simulink model "Pitch_Ap_testHarness"  (R2012b)
settings: Solver=FixedStepDiscrete  SolverMode=SingleTasking  StartTime=0  StopTime=0.25  FixedStep=0.025  RelTol=1e-3
model workspace (MAT data in the model file):
  dispGain = [3707764736; 2; 1; 1; 1; 1]
  intGain = [3707764736; 2; 1; 1; 2; 1]
  rateGain = [3707764736; 2; 1; 1; 3; 1]
undefined symbols (not defined in the file): sigbuilder_block
libraries: simulink x1
settings Model: SldvGeneratedHarnessModel=TestUnitModel=Pitch_Ap|  RecordCoverage=on  CovSaveName=covdata_pitchAP  CovMetricSettings=dcmoe  CovHTMLOptions=-aTS=1 -bRG=1 -bTC=0 -hTR=0 -nFC=0 -scm=1 -bcm=1  CovCumulativeVarName=covCumulativeData_pitchAP  CovCumulativeReport=on  CovReportOnPause=off  CovModelRefEnable=on  CovExternalEMLEnable=on  Creator=bpotter  LastModifiedBy=klindqvi
settings DataIOCC: LimitDataPoints=off  SaveFormat=StructureWithTime  SignalLoggingSaveFormat=ModelDataLogs  SaveOutput=off  DSMLogging=off  SaveTime=off  SignalLoggingName=logsOut
settings OptimizationCC: BlockReduction=off  InlineParams=on  UseIntDivNetSlope=on  InlineInvariantSignals=on  EnhancedBackFolding=on  ExpressionFolding=off  EnableMemcpy=off  PassReuseOutputArgsAs=Individual arguments  StateBitsets=on  DataBitsets=on  ZeroExternalMemoryAtStartup=off  ZeroInternalMemoryAtStartup=off  InitFltsAndDblsToZero=on  EfficientFloat2IntCast=on  EfficientMapNaN2IntZero=off  OptimizeModelRefInitCode=on  MaxStackSize=inf
settings DebuggingCC: SignalInfNanChecking=error  ReadBeforeWriteMsg=EnableAllAsError  WriteAfterWriteMsg=EnableAllAsError  WriteAfterReadMsg=EnableAllAsError  AlgebraicLoopMsg=error  ArtificialAlgebraicLoopMsg=error  SaveWithDisabledLinksMsg=error  SaveWithParameterizedLinksMsg=error  UnderspecifiedInitializationDetection=Simplified  BlockPriorityViolationMsg=error  MaxConsecutiveZCsMsg=warning  SolverPrmCheckMsg=error  InheritedTsInSrcMsg=none  DiscreteInheritContinuousMsg=error  SingleTaskRateTransMsg=error  TasksWithSamePriorityMsg=error  SigSpecEnsureSampleTimeMsg=error  CheckMatrixSingularityMsg=error  IntegerOverflowMsg=none  ParameterUnderflowMsg=error  ParameterPrecisionLossMsg=error  ParameterTunabilityLossMsg=error  UnderSpecifiedDataTypeMsg=error  UnnecessaryDatatypeConvMsg=warning  VectorMatrixConversionMsg=error  SignalLabelMismatchMsg=error  UnconnectedInputMsg=error  UnconnectedOutputMsg=error  UnconnectedLineMsg=error  SFcnCompatibilityMsg=error  UniqueDataStoreMsg=error  BusObjectLabelMismatch=error  RootOutportRequireBusObject=error  AssertControl=DisableAll  ModelReferenceIOMsg=error  ModelReferenceVersionMismatchMessage=warning  ModelReferenceIOMismatchMessage=error  UnknownTsInhSupMsg=error  ModelReferenceDataLoggingMessage=error  ModelReferenceExtraNoncontSigs=none  StrictBusMsg=ErrorOnBusTreatedAsVector  BusNameAdapt=ErrorWithoutRepair  NonBusSignalsTreatedAsBus=error
settings HardwareCC: ProdIntDivRoundTo=Zero  ProdEndianess=LittleEndian  ProdHWDeviceType=Specified
settings ModelReferenceCC: UpdateModelReferenceTargets=AssumeUpToDate  CheckModelReferenceTargetMessage=none
settings RTWCC: SystemTargetFile=ert.tlc  TemplateMakefile=ert_default_tmf  Description=Embedded Coder  GenerateReport=on  RTWVerbose=off  ProcessScript=ert_make_rtw_hook  IncludeHyperlinkInReport=on  GenerateTraceInfo=on  GenerateTraceReport=on  GenerateTraceReportSl=on  GenerateTraceReportSf=on  GenerateTraceReportEml=on  GenerateCodeMetricsReport=on
settings CodeAppCC: ForceParamTrailComments=on  IgnoreCustomStorageClasses=off  IgnoreTestpoints=on  SimulinkDataObjDesc=on  MangleLength=4  CustomSymbolStrGlobalVar=$N$M  CustomSymbolStrType=$N$M  CustomSymbolStrFcn=$N$M$F  CustomSymbolStrMacro=$N$M  InsertBlockDesc=on  ReqsInCode=on
settings ERTTargetCC: CodeReplacementLibrary=ANSI_C  UtilityFuncGeneration=Shared location  MultiwordLength=2048  GenerateSampleERTMain=on  IncludeMdlTerminateFcn=off  GeneratePreprocessorConditionals=Disable all  SuppressErrorStatus=on  SupportAbsoluteTime=off  MultiInstanceERTCode=on  SupportNonFinite=off  SupportComplex=off  ParenthesesLevel=Maximum  InlinedParameterPlacement=NonHierarchical  ERTCustomFileTemplate=example_file_process.tlc  ERTFilePackagingFormat=CompactWithDataFile  PreserveExpressionOrder=on  PreserveIfCondition=on  ConvertIfToSwitch=off  SuppressUnreachableDefaultCases=off

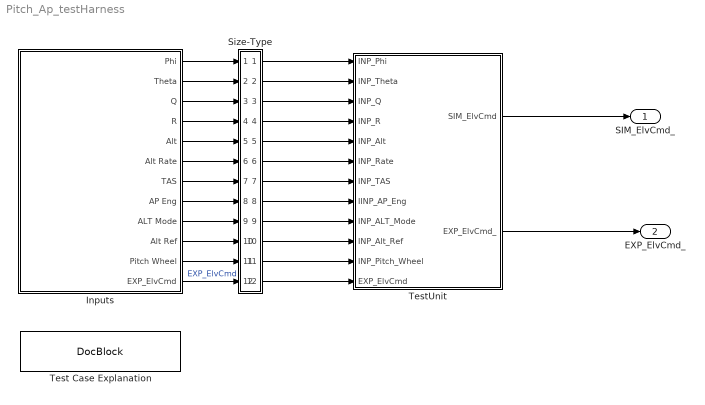
== system Pitch_Ap_testHarness ==
  Inputs : Subsystem  Tag=STV Subsys  LoadFcn=sigbuilder_block('load');  StartFcn=sigbuilder_block('start');  StopFcn=sigbuilder_block('stop');  ClipboardFcn=sigbuilder_block('clipboard');  mask(Sigbuilder block){}
      mask init:
      | if ~strcmp(get_param(bdroot(gcb),'SimulationStatus'),'stopped'),tuvar = sigbuilder_block('maskInit'); end
      settings: CopyFcn=sigbuilder_block('copy');  DeleteFcn=sigbuilder_block('delete');  ModelCloseFcn=sigbuilder_block('modelClose');  PreSaveFcn=sigbuilder_block('preSave');  PauseFcn=sigbuilder_block('pause');  ContinueFcn=sigbuilder_block('continue');  NameChangeFcn=sigbuilder_block('namechange');  OpenFcn=sigbuilder_block('open',[18 174 755.25 438 ]);  CloseFcn=sigbuilder_block('close');
      mask Display: plot(0, 0, 100, 100,[2, 2, 32, 32, 2], [68, 8, 8, 68, 68],[32, 2], [38, 38], [32, 19, 2],[53, 60, 44], [32, 17, 17, 2],[16, 16, 31, 31]);txt = getActiveGroup(gcbh);text(2, 100, txt,'verticalAlignment', 'top');
  Size-Type : Subsystem
  Test Case Explanation : simulink/Model-Wide Utilities/DocBlock  DocumentType=Text
      content=|
      | Test Case 1 (38 Objectives)
      | 	Parameter values:
      |
      | 	1. Altitude Mode/Rate Limiter/Saturation Dynamic/Switch - logical trigger input false (output is from 3rd input port) @ T=0.08
      | 	2. Altitude Mode/Rate Limiter/Saturation Dynamic/Switch - logical trigger input true (output is from 1st input port) @ T=0.15
      | 	3. Attitude_Controller/Cmd Limit - input > lower limit T @ T=0.05
      | 	4. Attitude_Controller/Cmd Limit - input >= upper limit F @ T=0.05
      | 	5. Attitude_Controller/LevelResetIntegrator/Saturation - input > lower limit T @ T=0.05
      | 	6. Attitude_Controller/LevelResetIntegrator/Saturation - input >= upper limit F @ T=0.05
      | 	7. Pitch Reference/Latch Theta/Enable - logical trigger input false (output is from 3rd input port) @ T=0.05
      | 	8. Pitch Reference/Latch Theta/Enable - logical trigger input true (output is from 1st input port) @ T=0.00
      | 	9. Altitude Mode/Rate Limiter/Saturation Dynamic/Switch2 - logical trigger input false (output is from 3rd input port) @ T=0.08
      | 	10. Altitude Mode/Rate Limiter/Saturation Dynamic/Switch2 - logical trigger input true (output is from 1st input port) @ T=0.00
      | 	11. Altitude Mode/Switch - logical trigger input false (output is from 3rd input port) @ T=0.10
      | 	12. Altitude Mode/Switch - logical trigger input true (output is from 1st input port) @ T=0.00
      | 	13. Attitude_Controller/LevelResetIntegrator/Switch1 - logical trigger input false (output is from 3rd input port) @ T=0.05
      | 	14. Attitude_Controller/LevelResetIntegrator/Switch1 - logical trigger input true (output is from 1st input port) @ T=0.00
      | 	15. Eng switch - logical trigger input false (output is from 3rd input port) @ T=0.00
      | 	16. Eng switch - logical trigger input true (output is from 1st input port) @ T=0.05
      | 	17. Mode switch - logical trigger input false (output is from 3rd input port) @ T=0.00
      | 	18. Mode switch - logical trigger input true (output is from 1st input port) @ T=0.10
      | 	19. Pitch Reference/Not engaged - Logic: input port 1 T @ T=0.05
      | 	20. Pitch Reference/Not engaged - Logic: input port 1 F @ T=0.00
      | 	21. Altitude Mode/Integrator - Reset F @ T=0.13
      | 	22. Altitude Mode/Integrator - Reset T @ T=0.03
      | 	23. Altitude Mode/Integrator - integration result <= lower limit F @ T=0.05
      | 	24. Altitude Mode/Integrator - integration result <= lower limit T @ T=0.00
      | 	25. Altitude Mode/Integrator - integration result >= upper limit F @ T=0.00
      | 	26. Altitude Mode/Integrator - integration result >= upper limit T @ T=0.18
      | 	27. Altitude Mode/Not ALT - Logic: input port 1 T @ T=0.10
      | 	28. Altitude Mode/Not ALT - Logic: input port 1 F @ T=0.00
      | 	29. Attitude_Controller/LevelResetIntegrator/Switch - logical trigger input false (output is from 3rd input port) @ T=0.05
      | 	30. Attitude_Controller/LevelResetIntegrator/Switch - logical trigger input true (output is from 1st input port) @ T=0.00
      | 	31. Attitude_Controller/Rate Limit - input > lower limit T @ T=0.00
      | 	32. Attitude_Controller/Rate Limit - input >= upper limit F @ T=0.00
      | 	33. Attitude_Controller/Rate Limit - input >= upper limit T @ T=0.18
      | 	34. Attitude_Controller/Disp Limit - input > lower limit T @ T=0.00
      | 	35. Attitude_Controller/Disp Limit - input >= upper limit F @ T=0.00
      | 	36. Attitude_Controller/Disp Limit - input >= upper limit T @ T=0.20
      | 	37. Attitude_Controller/Not engaged - Logic: input port 1 T @ T=0.05
      | 	38. Attitude_Controller/Not engaged - Logic: input port 1 F @ T=0.00
      |
      | Test Case 2 (3 Objectives)
      | 	Parameter values:
      |
      | 	1. Attitude_Controller/Cmd Limit - input > lower limit F @ T=0.00
      | 	2. Attitude_Controller/Rate Limit - input > lower limit F @ T=0.00
      | 	3. Attitude_Controller/Disp Limit - input > lower limit F @ T=0.03
      |
      | Test Case 3 (1 Objectives)
      | 	Parameter values:
      |
      | 	1. Attitude_Controller/Cmd Limit - input >= upper limit T @ T=0.00
  TestUnit : Subsystem
  SIM_ElvCmd_ : Outport  OutDataTypeStr=double  PortDimensions=1  SampleTime=1/40
  EXP_ElvCmd_ : Outport  Port=2  OutDataTypeStr=double  PortDimensions=1  SampleTime=1/40
  wires:
  Inputs/1(Phi) -> Size-Type/1(In1)
  Inputs/2(Theta) -> Size-Type/2(In2)
  Inputs/3(Q) -> Size-Type/3(In3)
  Inputs/4(R) -> Size-Type/4(In4)
  Inputs/5(Alt) -> Size-Type/5(In5)
  Inputs/6(Alt Rate) -> Size-Type/6(In6)
  Inputs/7(TAS) -> Size-Type/7(In7)
  Inputs/8(AP Eng) -> Size-Type/8(In8)
  Inputs/9(ALT Mode) -> Size-Type/9(In9)
  Inputs/10(Alt Ref) -> Size-Type/10(In10)
  Inputs/11("Pitch Wheel ") -> Size-Type/11(In11)
  Size-Type/1(Out1) -> TestUnit/1(INP_Phi)
  Size-Type/2(Out2) -> TestUnit/2(INP_Theta)
  Size-Type/3(Out3) -> TestUnit/3(INP_Q)
  Size-Type/4(Out4) -> TestUnit/4(INP_R)
  Size-Type/5(Out5) -> TestUnit/5(INP_Alt)
  Size-Type/6(Out6) -> TestUnit/6(INP_Rate)
  Size-Type/7(Out7) -> TestUnit/7(INP_TAS)
  Size-Type/8(Out8) -> TestUnit/8(IINP_AP_Eng)
  Size-Type/9(Out9) -> TestUnit/9(INP_ALT_Mode)
  Size-Type/10(Out10) -> TestUnit/10(INP_Alt_Ref)
  Size-Type/11(Out11) -> TestUnit/11(INP_Pitch_Wheel)
  TestUnit/1(SIM_ElvCmd) -> SIM_ElvCmd_/1
  TestUnit/2(EXP_ElvCmd_) -> EXP_ElvCmd_/1
  Inputs/12(EXP_ElvCmd) -> Size-Type/12(In12)  "EXP_ElvCmd"
  Size-Type/12(Out12) -> TestUnit/12(EXP_ElvCmd)

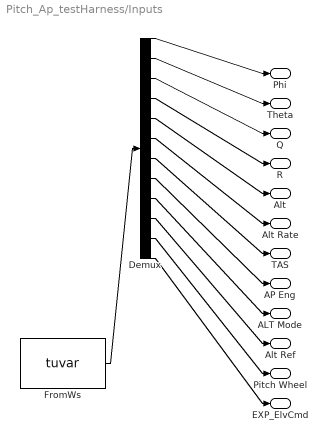
== system Pitch_Ap_testHarness/Inputs ==
  Demux : Demux  Tag=STV Demux  Outputs=12
  FromWs : FromWorkspace  Tag=STV FromWs  VariableName=tuvar  SampleTime=0
      SigBuilderData=|
      | dataSet(1).timeRange = [0 0.25]
      | dataSet(1).name = 'Test Case 1'
      | dataSet(2).timeRange = [0 0.075]
      | dataSet(2).name = 'Test Case 2'
      | dataSet(3).timeRange = [0 0.05]
      | dataSet(3).name = 'Test Case 3'
      | sbobj.Name = 'Signal Builder'
      | sbobj.Groups(1).Name = 'Test Case 1'
      | sbobj.Groups(1).Signals(1).Name = 'Phi'
      | sbobj.Groups(1).Signals(1).XData = [0 0.05 0.05 0.1 0.15 0.15 0.175 0.175 0.2 0.2 0.225 0.25]
      | sbobj.Groups(1).Signals(1).YData = [-8.54927 -8.54927 0 0 0 -6.7752 -6.7752 -1.37522 -1.37522 0 0 0]
      | sbobj.Groups(1).Signals(2).Name = 'Theta'
      | sbobj.Groups(1).Signals(2).XData = [0 0.05 0.05 0.1 0.1 0.15 0.15 0.175 0.175 0.2 0.2 0.225 0.225 0.25]
      | sbobj.Groups(1).Signals(2).YData = [0.8763 0.8763 0 0 0 0 1.88631 1.88631 -7.95353 -7.95353 0 0 0 0]
      | sbobj.Groups(1).Signals(3).Name = 'Q'
      | sbobj.Groups(1).Signals(3).XData = [0 0.05 0.05 0.1 0.1 0.15 0.15 0.175 0.175 0.2 0.2 0.225 0.225 0.25]
      | sbobj.Groups(1).Signals(3).YData = [9.81417 9.81417 0 0 0 0 4.66234 4.66234 3.21637 3.21637 0 0 0 0]
      | sbobj.Groups(1).Signals(4).Name = 'R'
      | sbobj.Groups(1).Signals(4).XData = [0 0.05 0.05 0.1 0.1 0.15 0.15 0.175 0.175 0.2 0.2 0.225 0.225 0.25]
      | sbobj.Groups(1).Signals(4).YData = [-5.97411 -5.97411 0 0 0 0 -2.73996 -2.73996 2.52191 2.52191 0 0 0 0]
      | sbobj.Groups(1).Signals(5).Name = 'Alt'
      | sbobj.Groups(1).Signals(5).XData = [0 0.05 0.05 0.1 0.1 0.15 0.15 0.175 0.175 0.2 0.2 0.225 0.225 0.25]
      | sbobj.Groups(1).Signals(5).YData = [3.08094 3.08094 0 0 0 0 -9.43223 -9.43223 -6.0138 -6.0138 0 0 0 0]
      | sbobj.Groups(1).Signals(6).Name = 'Alt Rate'
      | sbobj.Groups(1).Signals(6).XData = [0 0.05 0.05 0.1 0.1 0.15 0.15 0.175 0.175 0.2 0.2 0.225 0.225 0.25]
      | sbobj.Groups(1).Signals(6).YData = [2.41404 2.41404 0 0 0 0 -3.30183 -3.30183 5.00647 5.00647 0 0 0 0]
      | sbobj.Groups(1).Signals(7).Name = 'TAS'
      | sbobj.Groups(1).Signals(7).XData = [0 0.05 0.05 0.1 0.1 0.15 0.15 0.175 0.175 0.2 0.2 0.225 0.225 0.25]
      | sbobj.Groups(1).Signals(7).YData = [-1.71802 -1.71802 1 1 1 1 -6.6856 -6.6856 0.17805 0.17805 0.17805 0.17805 0.17805 0.17805]
      | sbobj.Groups(1).Signals(8).Name = 'AP Eng'
      | sbobj.Groups(1).Signals(8).XData = [0 0.05 0.05 0.1 0.1 0.15 0.15 0.175 0.175 0.2 0.2 0.225 0.225 0.25]
      | sbobj.Groups(1).Signals(8).YData = [0 0 1 1 0 0 0 0 0 0 0 0 0 0]
      | sbobj.Groups(1).Signals(9).Name = 'ALT Mode'
      | sbobj.Groups(1).Signals(9).XData = [0 0.05 0.05 0.1 0.1 0.15 0.15 0.175 0.175 0.2 0.2 0.225 0.225 0.25]
      | sbobj.Groups(1).Signals(9).YData = [0 0 0 0 1 1 1 1 0 0 0 0 0 0]
      | sbobj.Groups(1).Signals(10).Name = 'Alt Ref'
      | sbobj.Groups(1).Signals(10).XData = [0 0.05 0.05 0.1 0.1 0.15 0.15 0.175 0.175 0.2 0.2 0.225 0.225 0.25]
      | sbobj.Groups(1).Signals(10).YData = [-1.87545 -1.87545 0 0 0 0 1.18273 1.18273 -4.7876 -4.7876 0 0 0 0]
      | sbobj.Groups(1).Signals(11).Name = 'Pitch Wheel '
      | sbobj.Groups(1).Signals(11).XData = [0 0.05 0.05 0.1 0.1 0.15 0.15 0.175 0.175 0.2 0.2 0.225 0.225 0.25]
      | sbobj.Groups(1).Signals(11).YData = [0.54371 0.54371 0 0 0 0 1.80355 1.80355 -1.13153 -1.13153 27.95353 27.95353 27.95353 27.95353]
      | sbobj.Groups(1).Signals(12).Name = 'EXP_ElvCmd'
      | sbobj.Groups(1).Signals(12).XData = [0 0.025 0.05 0.075 0.1 0.125 0.15 0.175 0.2 0.225 0.25]
      | sbobj.Groups(1).Signals(12).YData = [0 0 2.6289 2.6508075 0 0 0 0 0 0 0]
      | sbobj.Groups(1).TimeRange = [0 0.25]
      | sbobj.Groups(2).Name = 'Test Case 2'
      | sbobj.Groups(2).Signals(1).Name = 'Phi'
      | sbobj.Groups(2).Signals(1).XData = [0 0.025 0.025 0.05 0.075]
      | sbobj.Groups(2).Signals(1).YData = [-2.89417 -2.89417 0 0 0]
      | sbobj.Groups(2).Signals(2).Name = 'Theta'
      | sbobj.Groups(2).Signals(2).XData = [0 0.025 0.025 0.05 0.075]
      | sbobj.Groups(2).Signals(2).YData = [-3.73326 -3.73326 0 0 0]
      | sbobj.Groups(2).Signals(3).Name = 'Q'
      | sbobj.Groups(2).Signals(3).XData = [0 0.025 0.025 0.05 0.075]
      | sbobj.Groups(2).Signals(3).YData = [3.93408 3.93408 0 0 0]
      | sbobj.Groups(2).Signals(4).Name = 'R'
      | sbobj.Groups(2).Signals(4).XData = [0 0.025 0.025 0.05 0.075]
      | sbobj.Groups(2).Signals(4).YData = [-9.33347 -9.33347 0 0 0]
      | sbobj.Groups(2).Signals(5).Name = 'Alt'
      | sbobj.Groups(2).Signals(5).XData = [0 0.025 0.025 0.05 0.075]
      | sbobj.Groups(2).Signals(5).YData = [-6.11826 -6.11826 0 0 0]
      | sbobj.Groups(2).Signals(6).Name = 'Alt Rate'
      | sbobj.Groups(2).Signals(6).XData = [0 0.025 0.025 0.05 0.075]
      | sbobj.Groups(2).Signals(6).YData = [-2.65354 -2.65354 0 0 0]
      | sbobj.Groups(2).Signals(7).Name = 'TAS'
      | sbobj.Groups(2).Signals(7).XData = [0 0.025 0.05 0.075]
      | sbobj.Groups(2).Signals(7).YData = [-8.84989 -8.84989 -8.84989 -8.84989]
      | sbobj.Groups(2).Signals(8).Name = 'AP Eng'
      | sbobj.Groups(2).Signals(8).XData = [0 0.025 0.025 0.05 0.075]
      | sbobj.Groups(2).Signals(8).YData = [1 1 0 0 0]
      | sbobj.Groups(2).Signals(9).Name = 'ALT Mode'
      | sbobj.Groups(2).Signals(9).XData = [0 0.025 0.05 0.075]
      | sbobj.Groups(2).Signals(9).YData = [0 0 0 0]
      | sbobj.Groups(2).Signals(10).Name = 'Alt Ref'
      | sbobj.Groups(2).Signals(10).XData = [0 0.025 0.025 0.05 0.075]
      | sbobj.Groups(2).Signals(10).YData = [-5.26616 -5.26616 0 0 0]
      | sbobj.Groups(2).Signals(11).Name = 'Pitch Wheel '
      | sbobj.Groups(2).Signals(11).XData = [0 0.025 0.025 0.05 0.075]
      | sbobj.Groups(2).Signals(11).YData = [-7.90382 -7.90382 -20 -20 -20]
      | sbobj.Groups(2).Signals(12).Name = 'EXP_ElvCmd'
      | sbobj.Groups(2).Signals(12).XData = [0 0.025 0.05 0.075 0.1 0.125 0.15 0.175 0.2 0.225 0.25]
      | sbobj.Groups(2).Signals(12).YData = [-20 0 0 0 0 0 0 0 0 0 0]
      | sbobj.Groups(2).TimeRange = [0 0.075]
      | sbobj.Groups(3).Name = 'Test Case 3'
      | sbobj.Groups(3).Signals(1).Name = 'Phi'
      | sbobj.Groups(3).Signals(1).XData = [0 0.025 0.05]
      | sbobj.Groups(3).Signals(1).YData = [1.69356 1.69356 1.69356]
      | sbobj.Groups(3).Signals(2).Name = 'Theta'
      | sbobj.Groups(3).Signals(2).XData = [0 0.025 0.025 0.05]
      | sbobj.Groups(3).Signals(2).YData = [0 0 0 0]
      | sbobj.Groups(3).Signals(3).Name = 'Q'
      | sbobj.Groups(3).Signals(3).XData = [0 0.025 0.025 0.05]
      | sbobj.Groups(3).Signals(3).YData = [-9.67089102533 -9.67089102533 -9.67089102533 -9.67089102533]
      | sbobj.Groups(3).Signals(4).Name = 'R'
      | sbobj.Groups(3).Signals(4).XData = [0 0.025 0.025 0.05]
      | sbobj.Groups(3).Signals(4).YData = [0 0 0 0]
      | sbobj.Groups(3).Signals(5).Name = 'Alt'
      | sbobj.Groups(3).Signals(5).XData = [0 0.025 0.025 0.05]
      | sbobj.Groups(3).Signals(5).YData = [0 0 0 0]
      | sbobj.Groups(3).Signals(6).Name = 'Alt Rate'
      | sbobj.Groups(3).Signals(6).XData = [0 0.025 0.025 0.05]
      | sbobj.Groups(3).Signals(6).YData = [0 0 0 0]
      | sbobj.Groups(3).Signals(7).Name = 'TAS'
      | sbobj.Groups(3).Signals(7).XData = [0 0.025 0.025 0.05]
      | sbobj.Groups(3).Signals(7).YData = [-3.79583 -3.79583 -3.79583 -3.79583]
      | sbobj.Groups(3).Signals(8).Name = 'AP Eng'
      | sbobj.Groups(3).Signals(8).XData = [0 0.025 0.025 0.05]
      | sbobj.Groups(3).Signals(8).YData = [1 1 1 1]
      | sbobj.Groups(3).Signals(9).Name = 'ALT Mode'
      | sbobj.Groups(3).Signals(9).XData = [0 0.025 0.025 0.05]
      | sbobj.Groups(3).Signals(9).YData = [0 0 0 0]
      | sbobj.Groups(3).Signals(10).Name = 'Alt Ref'
      | sbobj.Groups(3).Signals(10).XData = [0 0.025 0.025 0.05]
      | sbobj.Groups(3).Signals(10).YData = [0 0 0 0]
      | sbobj.Groups(3).Signals(11).Name = 'Pitch Wheel '
      | sbobj.Groups(3).Signals(11).XData = [0 0.025 0.025 0.05]
      | sbobj.Groups(3).Signals(11).YData = [0 0 0 0]
      | sbobj.Groups(3).Signals(12).Name = 'EXP_ElvCmd'
      | sbobj.Groups(3).Signals(12).XData = [0 0.025 0.05 0.075 0.1 0.125 0.15 0.175 0.2 0.225 0.25]
      | sbobj.Groups(3).Signals(12).YData = [20 20 20 20 20 20 20 20 20 20 20]
      | sbobj.Groups(3).TimeRange = [0 0.05]
  Phi : Outport  Tag=STV Outport
  Theta : Outport  Tag=STV Outport  Port=2
  Q : Outport  Tag=STV Outport  Port=3
  R : Outport  Tag=STV Outport  Port=4
  Alt : Outport  Tag=STV Outport  Port=5
  Alt Rate : Outport  Tag=STV Outport  Port=6
  TAS : Outport  Tag=STV Outport  Port=7
  AP Eng : Outport  Tag=STV Outport  Port=8
  ALT Mode : Outport  Tag=STV Outport  Port=9
  Alt Ref : Outport  Tag=STV Outport  Port=10
  "Pitch Wheel " : Outport  Tag=STV Outport  Port=11
  EXP_ElvCmd : Outport  Tag=STV Outport  Port=12
  wires:
  FromWs/1 -> Demux/1
  Demux/1 -> Phi/1
  Demux/2 -> Theta/1
  Demux/3 -> Q/1
  Demux/4 -> R/1
  Demux/5 -> Alt/1
  Demux/6 -> Alt Rate/1
  Demux/7 -> TAS/1
  Demux/8 -> AP Eng/1
  Demux/9 -> ALT Mode/1
  Demux/10 -> Alt Ref/1
  Demux/11 -> "Pitch Wheel "/1
  Demux/12 -> EXP_ElvCmd/1

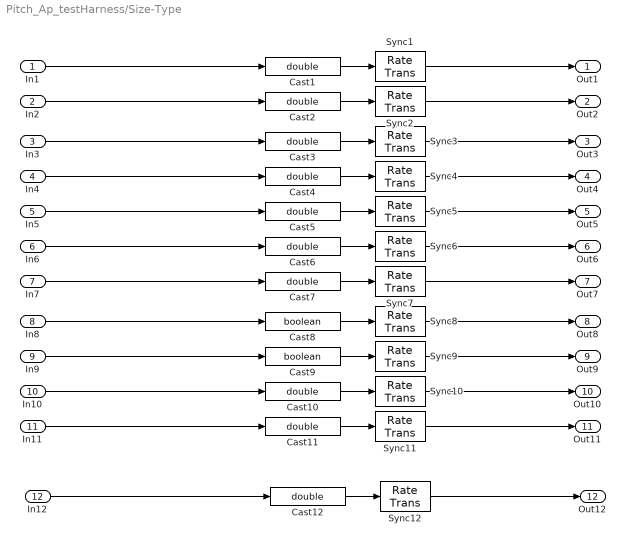
== system Pitch_Ap_testHarness/Size-Type ==
  In1 : Inport
  In2 : Inport  Port=2
  In3 : Inport  Port=3
  In4 : Inport  Port=4
  In5 : Inport  Port=5
  In6 : Inport  Port=6
  In7 : Inport  Port=7
  In8 : Inport  Port=8
  In9 : Inport  Port=9
  In10 : Inport  Port=10
  In11 : Inport  Port=11
  In12 : Inport  Port=12
  Cast{1..7,10..12} (10 alike) : DataTypeConversion  OutDataTypeStr=double  SaturateOnIntegerOverflow=on  RndMeth=Zero
  Cast8 : DataTypeConversion  OutDataTypeStr=boolean  SaturateOnIntegerOverflow=on  RndMeth=Zero
  Cast9 : DataTypeConversion  OutDataTypeStr=boolean  SaturateOnIntegerOverflow=on  RndMeth=Zero
  Sync{1..12} (12 alike) : RateTransition  OutPortSampleTime=[0.025000000000000001,0]
  Out1 : Outport
  Out2 : Outport  Port=2
  Out3 : Outport  Port=3
  Out4 : Outport  Port=4
  Out5 : Outport  Port=5
  Out6 : Outport  Port=6
  Out7 : Outport  Port=7
  Out8 : Outport  Port=8
  Out9 : Outport  Port=9
  Out10 : Outport  Port=10
  Out11 : Outport  Port=11
  Out12 : Outport  Port=12
  wires:
  In1/1 -> Cast1/1
  Cast1/1 -> Sync1/1
  Sync1/1 -> Out1/1
  In2/1 -> Cast2/1
  Cast2/1 -> Sync2/1
  Sync2/1 -> Out2/1
  In3/1 -> Cast3/1
  Cast3/1 -> Sync3/1
  Sync3/1 -> Out3/1
  In4/1 -> Cast4/1
  Cast4/1 -> Sync4/1
  Sync4/1 -> Out4/1
  In5/1 -> Cast5/1
  Cast5/1 -> Sync5/1
  Sync5/1 -> Out5/1
  In6/1 -> Cast6/1
  Cast6/1 -> Sync6/1
  Sync6/1 -> Out6/1
  In7/1 -> Cast7/1
  Cast7/1 -> Sync7/1
  Sync7/1 -> Out7/1
  In8/1 -> Cast8/1
  Cast8/1 -> Sync8/1
  Sync8/1 -> Out8/1
  In9/1 -> Cast9/1
  Cast9/1 -> Sync9/1
  Sync9/1 -> Out9/1
  In10/1 -> Cast10/1
  Cast10/1 -> Sync10/1
  Sync10/1 -> Out10/1
  In11/1 -> Cast11/1
  Cast11/1 -> Sync11/1
  Sync11/1 -> Out11/1
  In12/1 -> Cast12/1
  Cast12/1 -> Sync12/1
  Sync12/1 -> Out12/1

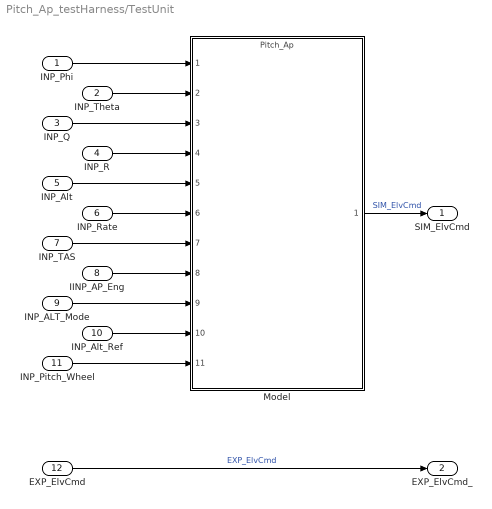
== system Pitch_Ap_testHarness/TestUnit ==
  INP_Phi : Inport
  INP_Theta : Inport  Port=2
  INP_Q : Inport  Port=3
  INP_R : Inport  Port=4
  INP_Alt : Inport  Port=5
  INP_Rate : Inport  Port=6
  INP_TAS : Inport  Port=7
  IINP_AP_Eng : Inport  Port=8
  INP_ALT_Mode : Inport  Port=9
  INP_Alt_Ref : Inport  Port=10
  INP_Pitch_Wheel : Inport  Port=11
  EXP_ElvCmd : Inport  Port=12
  Model : ModelReference  ModelNameDialog=Pitch_Ap  ParameterArgumentNames=dispGain,intGain,rateGain  ParameterArgumentValues=2 0.5 2  SimulationMode=Normal  ModelReferenceVersion=1.97  CopyOfModelName=Pitch_Ap  DefaultDataLogging=on
  SIM_ElvCmd : Outport
  EXP_ElvCmd_ : Outport  Port=2
  wires:
  INP_Phi/1 -> Model/1
  INP_Theta/1 -> Model/2
  INP_Q/1 -> Model/3
  INP_R/1 -> Model/4
  INP_Alt/1 -> Model/5
  INP_Rate/1 -> Model/6
  INP_TAS/1 -> Model/7
  IINP_AP_Eng/1 -> Model/8
  INP_ALT_Mode/1 -> Model/9
  INP_Alt_Ref/1 -> Model/10
  INP_Pitch_Wheel/1 -> Model/11
  Model/1 -> SIM_ElvCmd/1  "SIM_ElvCmd"
  EXP_ElvCmd/1 -> EXP_ElvCmd_/1  "EXP_ElvCmd"
